simulink model "exm2_4"  (Simulink 3.00)
settings: Solver=VariableStepDiscrete  SolverMode=SingleTasking  StartTime=0.0  StopTime=10.0  RelTol=1e-3  AbsTol=1e-6
settings Model: RTWTemplateMakefile=grt_vc.tmf

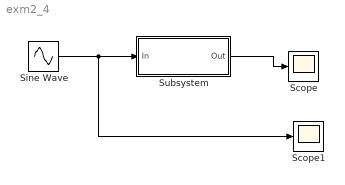
== system exm2_4 ==
  Scope : Scope
      settings: TickLabels=on  TimeRange=auto  YMin=-5  YMax=5  SaveToWorkspace=off  SaveName=ScopeData  DataFormat=Matrix
  Scope1 : Scope
      settings: TickLabels=on  TimeRange=auto  YMin=-5  YMax=5  SaveToWorkspace=off  SaveName=ScopeData  DataFormat=Matrix
  Sine Wave : Sin  Amplitude=1  Frequency=1  Phase=0  SampleTime=0
  Subsystem : Subsystem  mask(comparater){th=0.5}
      mask prompts: th "threshold"
      mask Display: disp('The Comparater')
  wires:
  Subsystem/1(Out) -> Scope/1
  Sine Wave/1 -> Subsystem/1(In), Scope1/1

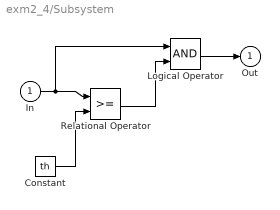
== system exm2_4/Subsystem ==
  In : Inport  Port=1  PortWidth=-1  SampleTime=-1  DataType=auto
      settings: SignalType=auto
  Constant : Constant  Value=th
  Logical Operator : Logic  Operator=AND  Inputs=2
  Relational Operator : RelationalOperator  Operator=>=
  Out : Outport  Port=1  InitialOutput=0
  wires:
  Relational Operator/1 -> Logical Operator/2
  Constant/1 -> Relational Operator/2
  In/1 -> Relational Operator/1, Logical Operator/1
  Logical Operator/1 -> Out/1
